simulink model "EXPERIMENT_01_RL_030x5B10x5D"  (R2023b)
settings: Solver=VariableStepAuto  StartTime=0.0  StopTime=.2  RelTol=1e-3
libraries: spsRMSLib x4, spsPowerLib x3, spsVoltageMeasurementLib x3, spsSeriesRLCBranchLib x2, spsACVoltageSourceLib x1, spsCurrentMeasurementLib x1, sps_lib x1
settings Model: Creator=deves  LastModifiedBy=ASUS

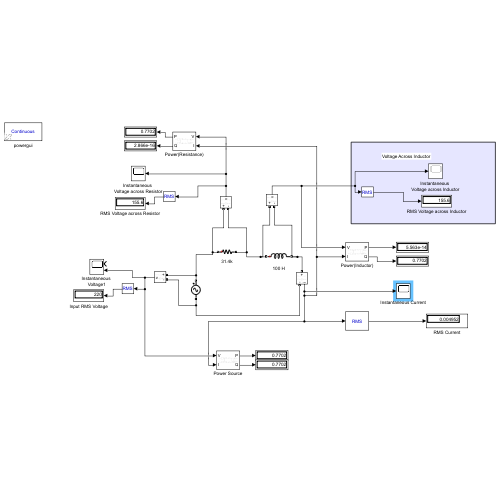
[thumbnail: Simulink's stored preview of the top-level diagram]
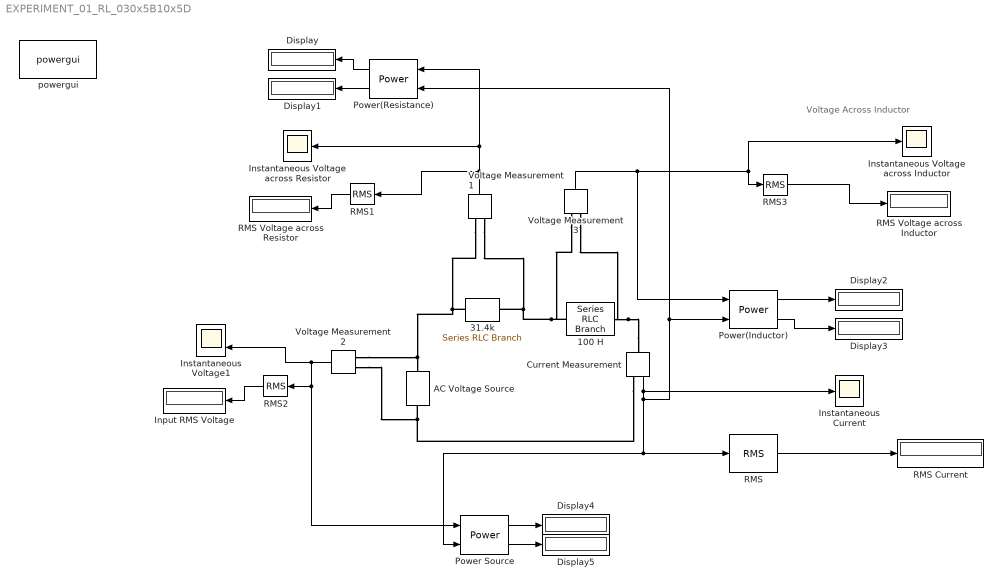
== system EXPERIMENT_01_RL_030x5B10x5D ==
  note: Voltage Across Inductor
  100 H : spsSeriesRLCBranchLib/Series RLC Branch  LConnTagsString=__new0  RConnTagsString=__new0  BranchType=L  Resistance=1  Inductance=100  SetiL0=off  InitialCurrent=0  Capacitance=1e-6  Setx0=off  InitialVoltage=0  Measurements=None
  31.4k : spsSeriesRLCBranchLib/Series RLC Branch  LConnTagsString=__new0  RConnTagsString=__new0  BranchType=R  Resistance=10*pi*10^3  Inductance=1e-3  SetiL0=off  InitialCurrent=0  Capacitance=1e-6  Setx0=off  InitialVoltage=0  Measurements=None
  AC Voltage Source : spsACVoltageSourceLib/AC Voltage Source  Amplitude=220*(sqrt(2))  Phase=0  Frequency=50  SampleTime=0.0001  Measurements=Voltage  BusType=swing  Pref=10e3  Qref=0  Qmin=-inf  Qmax=+inf
  Current Measurement : spsCurrentMeasurementLib/Current Measurement  PhasorSimulation=off  OutputType=Complex  PSBequivalent=0
  Display{,1..5} (6 alike) : Display
  Input RMS Voltage : Display
  Instantaneous Voltage across Inductor : Scope
  Instantaneous Voltage across Resistor : Scope
  Instantaneous Voltage1 : Scope  NumInputPorts=2
  Instantaneous Current : Scope
  Power Source : spsPowerLib/Power  Freq=50  Vinit=[1, 0]  Iinit=[1, 0]  Ts=0
  Power(Inductor) : spsPowerLib/Power  Freq=50  Vinit=[1, 0]  Iinit=[1, 0]  Ts=0
  Power(Resistance) : spsPowerLib/Power  Freq=50  Vinit=[1, 0]  Iinit=[1, 0]  Ts=0
  RMS{,1..3} (4 alike) : spsRMSLib/RMS  TrueRMS=on  Freq=50  RMSInit=120  Ts=0
  RMS Current : Display
  RMS Voltage across Inductor : Display
  RMS Voltage across Resistor : Display
  Voltage Measurement1 : spsVoltageMeasurementLib/Voltage Measurement  PhasorSimulation=off  OutputType=Complex  PSBequivalent=0
  Voltage Measurement2 : spsVoltageMeasurementLib/Voltage Measurement  PhasorSimulation=off  OutputType=Complex  PSBequivalent=0
  Voltage Measurement3 : spsVoltageMeasurementLib/Voltage Measurement  PhasorSimulation=off  OutputType=Complex  PSBequivalent=0
  powergui : sps_lib/powergui  Priority=1  SimulationMode=Continuous  SampleTime=50e-6  frequency=60  Iterations=50  frequencyindice=50  Pbase=100e6  ErrMax=1e-4  UnitsV=kV  UnitsW=MW  buscounter=0  FunctionMessages=off  echomessages=off  EnableUseOfTLC=off  CurrentSourceSwitches=off  DisableSnubberDevices=off  DisableRonSwitches=off  DisableVfSwitches=off  DisplayEquations=off  AutomaticDiscreteSolvers=off  SolverType=Tustin/Backward Euler (TBE)  Interpol=off  ExternalGateDelay=off  methode=off  Ts=100  x0status=blocks  SPID=on  SwTol=0  HookPort=off  NonlinearTolerance=1e-4  nMaxIteration=100  ContinueOnMaxIteration=off  RestoreLinks=warning  ResistiveCurrentMeasurement=off  Frange=[0:2:500]  Ylog=off  Xlog=on  ShowGrid=off  save=off  variable=ZData  structure=0  ZoomFFT=off  StartTime=0.0  cycles=1  DisplayStyle=1  fundamental=60  FreqAxis=off  MaxFrequency=1000  frequencyindicesteady=1  RmsSteady=1  display=off
  wires:
  Voltage Measurement1/1 -> Power(Resistance)/1, Instantaneous Voltage across Resistor/1, RMS1/1
  RMS/1 -> RMS Current/1
  Voltage Measurement3/1 -> Power(Inductor)/1, RMS3/1, Instantaneous Voltage across Inductor/1
  Power(Resistance)/1 -> Display/1
  RMS3/1 -> RMS Voltage across Inductor/1
  RMS2/1 -> Input RMS Voltage/1
  RMS1/1 -> RMS Voltage across Resistor/1
  Power(Inductor)/2 -> Display3/1
  Power(Inductor)/1 -> Display2/1
  Power(Resistance)/2 -> Display1/1
  Current Measurement/1 -> Power(Inductor)/2, Power(Resistance)/2, RMS/1, Power Source/2, Instantaneous Current/1
  Power Source/1 -> Display4/1
  Voltage Measurement2/1 -> Power Source/1, RMS2/1, Instantaneous Voltage1/2
  Power Source/2 -> Display5/1
  connections:
  AC Voltage Source/RConn1 -- Voltage Measurement2/LConn1 -- Voltage Measurement1/LConn1 -- 31.4k/LConn1
  Current Measurement/LConn1 -- 100 H/RConn1 -- Voltage Measurement3/LConn2
  31.4k/RConn1 -- Voltage Measurement1/LConn2 -- 100 H/LConn1 -- Voltage Measurement3/LConn1
  AC Voltage Source/LConn1 -- Current Measurement/RConn1 -- Voltage Measurement2/LConn2
